simulink model "six_bots_Observer_Collision_MN_VP_NAPF"  (R2021a)
settings: Solver=ode5  StartTime=0.0  StopTime=20  FixedStep=0.005  RelTol=1e-3
(part 1 of 4)
settings Model: Creator=a1752760  LastModifiedBy=a1752760
settings SolverCC: AlgebraicLoopSolver=TrustRegion
settings DataIOCC: ReturnWorkspaceOutputs=off
settings DebuggingCC: SFMachineParentedDataDiag=warning  ArithmeticOperatorsInVariantConditions=warning
settings SFSimCC: CustomCodeUndefinedFunction=UseInterfaceOnly

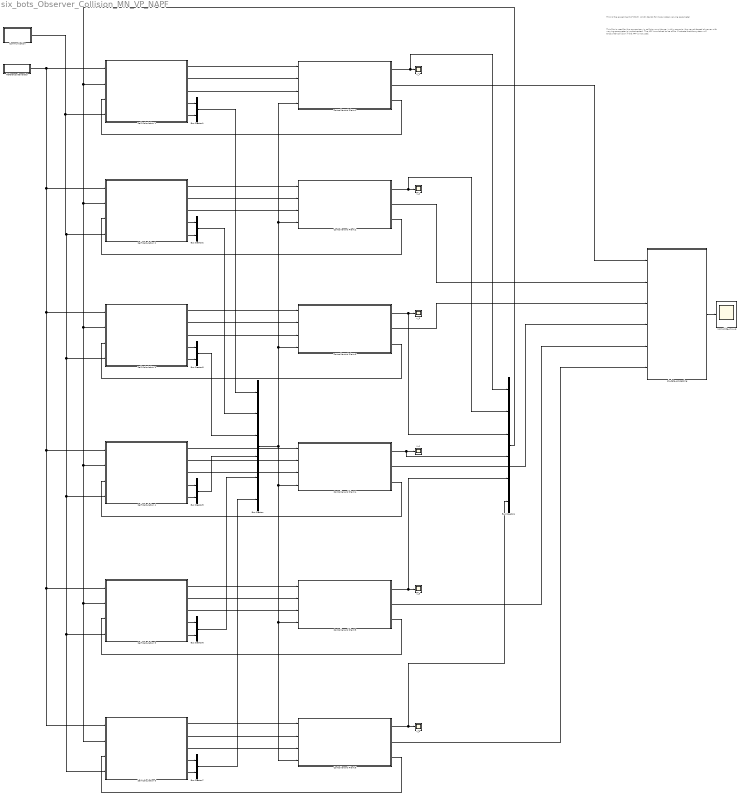
== system six_bots_Observer_Collision_MN_VP_NAPF ==
  note: This file is used for the comparison in collision avoidance. In this scenario, the neural-based
      | observer with varying-parameter is implemented. The APF is switched to be off to illustrate
      | that the system will encounter collision if the APF is not used.
  note: This is the experiment of MNVP, which stands for more nodes varying parameter
  Bus Creator : BusCreator  Inputs=6
  Bus Creator{1..3,5..7} (6 alike) : BusCreator  Inputs=2
  Bus Creator4 : BusCreator  Inputs=6
  Communication : Subsystem
  Controller and Plant 1 : Subsystem  mask{x_1=[1.8;0.1;0]}
      mask prompts: x_1 "Simulink:blkprm_prompts:IntegratorInitCond"
      mask TypeOptions x_1: x_1/InitialCondition
      mask DialogControl x_1 Prompt: Initial condition:
  Controller and Plant 2 : Subsystem  mask{x_2=[-0.9;0.6;pi/3]}
      mask prompts: x_2 "Simulink:blkprm_prompts:IntegratorInitCond"
      mask TypeOptions x_2: x_2/InitialCondition
      mask DialogControl x_2 Prompt: Initial condition:
  Controller and Plant 3 : Subsystem  mask{x_3=[-0.7;2.3;-pi/3]}
      mask prompts: x_3 "Simulink:blkprm_prompts:IntegratorInitCond"
      mask TypeOptions x_3: x_3/InitialCondition
      mask DialogControl x_3 Prompt: Initial condition:
  Controller and Plant 4 : Subsystem  mask{x_4=[0.8;-0.5;pi/2]}
      mask prompts: x_4 "Simulink:blkprm_prompts:IntegratorInitCond"
      mask TypeOptions x_4: x_4/InitialCondition
      mask DialogControl x_4 Prompt: Initial condition:
  Controller and Plant 5 : Subsystem  mask{x_5=[-0.1;-1.3;pi/4]}
      mask prompts: x_5 "Simulink:blkprm_prompts:IntegratorInitCond"
      mask TypeOptions x_5: x_5/InitialCondition
      mask DialogControl x_5 Prompt: Initial condition:
  Controller and Plant 6 : Subsystem  mask{x_6=[1.5;1.5;-pi/4]}
      mask prompts: x_6 "Simulink:blkprm_prompts:IntegratorInitCond"
      mask TypeOptions x_6: x_6/InitialCondition
      mask DialogControl x_6 Prompt: Initial condition:
  Reference Generator : Subsystem
  Self Calculation 1 : Subsystem
  Self Calculation 2 : Subsystem
  Self Calculation 3 : Subsystem
  Self Calculation 4 : Subsystem
  Self Calculation 5 : Subsystem
  Self Calculation 6 : Subsystem
  norm_tilde_mn_vp : Scope
  ob_data_processing : MATLAB Function  TreatAsAtomicUnit=on
  x_{1..6} (6 alike) : Scope
  wires:
  Controller and Plant 1/1(Position_1) -> Bus Creator4/1, x_1/1
  Controller and Plant 1/3(Control input_1) -> Self Calculation 1/3(Control Input)
  Self Calculation 1/4(delta_x) -> Bus Creator1/1
  Self Calculation 1/5(delta_v) -> Bus Creator1/2
  Self Calculation 1/1(L_i) -> Controller and Plant 1/1(L_i)
  Self Calculation 1/2(u_bar) -> Controller and Plant 1/2(u_bar)
  Self Calculation 1/3(Z_1) -> Controller and Plant 1/3(Z_1)
  Self Calculation 2/3(Z_1) -> Controller and Plant 2/3(Z_1)
  Self Calculation 2/4(delta_x) -> Bus Creator2/1
  Self Calculation 2/1(L_i) -> Controller and Plant 2/1(L_i)
  Controller and Plant 2/3(Control input_1) -> Self Calculation 2/3(Control Input)
  Self Calculation 2/2(u_bar) -> Controller and Plant 2/2(u_bar)
  Self Calculation 2/5(delta_v) -> Bus Creator2/2
  Self Calculation 3/3(Z_1) -> Controller and Plant 3/3(Z_1)
  Self Calculation 3/4(delta_x) -> Bus Creator3/1
  Self Calculation 3/1(L_i) -> Controller and Plant 3/1(L_i)
  Controller and Plant 3/3(Control input_1) -> Self Calculation 3/3(Control Input)
  Self Calculation 3/2(u_bar) -> Controller and Plant 3/2(u_bar)
  Self Calculation 3/5(delta_v) -> Bus Creator3/2
  Controller and Plant 2/1(Position_1) -> Bus Creator4/2, x_2/1
  Controller and Plant 3/1(Position_1) -> Bus Creator4/3, x_3/1
  Controller and Plant 4/3(Control input_1) -> Self Calculation 4/3(Control Input)
  Controller and Plant 4/1(Position_1) -> Bus Creator4/4, x_4/1
  Self Calculation 4/5(delta_v) -> Bus Creator5/2
  Self Calculation 4/2(u_bar) -> Controller and Plant 4/2(u_bar)
  Self Calculation 4/3(Z_1) -> Controller and Plant 4/3(Z_1)
  Self Calculation 4/4(delta_x) -> Bus Creator5/1
  Self Calculation 4/1(L_i) -> Controller and Plant 4/1(L_i)
  Controller and Plant 5/3(Control input_1) -> Self Calculation 5/3(Control Input)
  Self Calculation 5/5(delta_v) -> Bus Creator6/2
  Self Calculation 5/2(u_bar) -> Controller and Plant 5/2(u_bar)
  Self Calculation 5/3(Z_1) -> Controller and Plant 5/3(Z_1)
  Self Calculation 5/4(delta_x) -> Bus Creator6/1
  Self Calculation 5/1(L_i) -> Controller and Plant 5/1(L_i)
  Controller and Plant 6/3(Control input_1) -> Self Calculation 6/3(Control Input)
  Controller and Plant 6/1(Position_1) -> Bus Creator4/6, x_6/1
  Self Calculation 6/5(delta_v) -> Bus Creator7/2
  Self Calculation 6/2(u_bar) -> Controller and Plant 6/2(u_bar)
  Self Calculation 6/3(Z_1) -> Controller and Plant 6/3(Z_1)
  Self Calculation 6/4(delta_x) -> Bus Creator7/1
  Communication/1(Laplacian) -> Self Calculation 2/4(Laplacian), Self Calculation 6/4(Laplacian), Self Calculation 5/4(Laplacian), Self Calculation 4/4(Laplacian), Self Calculation 3/4(Laplacian), Self Calculation 1/4(Laplacian)
  Reference Generator/1(Full_reference) -> Self Calculation 2/1(Reference), Self Calculation 6/1(Reference), Self Calculation 5/1(Reference), Self Calculation 4/1(Reference), Self Calculation 3/1(Reference), Self Calculation 1/1(Reference)
  Self Calculation 6/1(L_i) -> Controller and Plant 6/1(L_i)
  Bus Creator1/1 -> Bus Creator/1
  Bus Creator2/1 -> Bus Creator/2
  Bus Creator3/1 -> Bus Creator/3
  Bus Creator5/1 -> Bus Creator/4
  Bus Creator6/1 -> Bus Creator/5
  Bus Creator7/1 -> Bus Creator/6
  Controller and Plant 5/1(Position_1) -> Bus Creator4/5, x_5/1
  Bus Creator4/1 -> Self Calculation 6/2(Position_agents), Self Calculation 5/2(Position_agents), Self Calculation 4/2(Position_agents), Self Calculation 3/2(Position_agents), Self Calculation 2/2(Position_agents), Self Calculation 1/2(Position_agents)
  Bus Creator/1 -> Controller and Plant 3/4(info_commu), Controller and Plant 2/4(info_commu), Controller and Plant 1/4(info_commu), Controller and Plant 6/4(info_commu), Controller and Plant 5/4(info_commu), Controller and Plant 4/4(info_commu)
  Controller and Plant 1/2(ob_tilde_1) -> ob_data_processing/1(ob_tilde_1)
  Controller and Plant 2/2(ob_tilde_2) -> ob_data_processing/2(ob_tilde_2)
  Controller and Plant 3/2(ob_tilde_3) -> ob_data_processing/3(ob_tilde_3)
  Controller and Plant 4/2(ob_tilde_4) -> ob_data_processing/4(ob_tilde_4)
  Controller and Plant 5/2(ob_tilde_5) -> ob_data_processing/5(ob_tilde_5)
  Controller and Plant 6/2(ob_tilde_6) -> ob_data_processing/6(ob_tilde_6)
  ob_data_processing/1(norm_tilde) -> norm_tilde_mn_vp/1

== system six_bots_Observer_Collision_MN_VP_NAPF/Communication ==
  Add : Sum
  Communication Topology : Constant  Value=[1,-1,0,0,0,0;0,1,-1,0,0,0;-1,-1,3,0,0,-1;0,0,-1,2,-1,0;0,0,0,0,1,-1;0,0,-1,-1,0,2]  VectorParams1D=off
  Constant : Constant  Value=2  VectorParams1D=off
  Product : Product
  Reference Feeding : Constant  Value=[1,0,0,0,0,0;0,1,0,0,0,0;0,0,1,0,0,0;0,0,0,1,0,0;0,0,0,0,1,0;0,0,0,0,0,1]  VectorParams1D=off
  Laplacian : Outport  VectorParamsAs1DForOutWhenUnconnected=off
  wires:
  Constant/1 -> Product/2
  Reference Feeding/1 -> Product/1
  Communication Topology/1 -> Add/1
  Product/1 -> Add/2
  Add/1 -> Laplacian/1

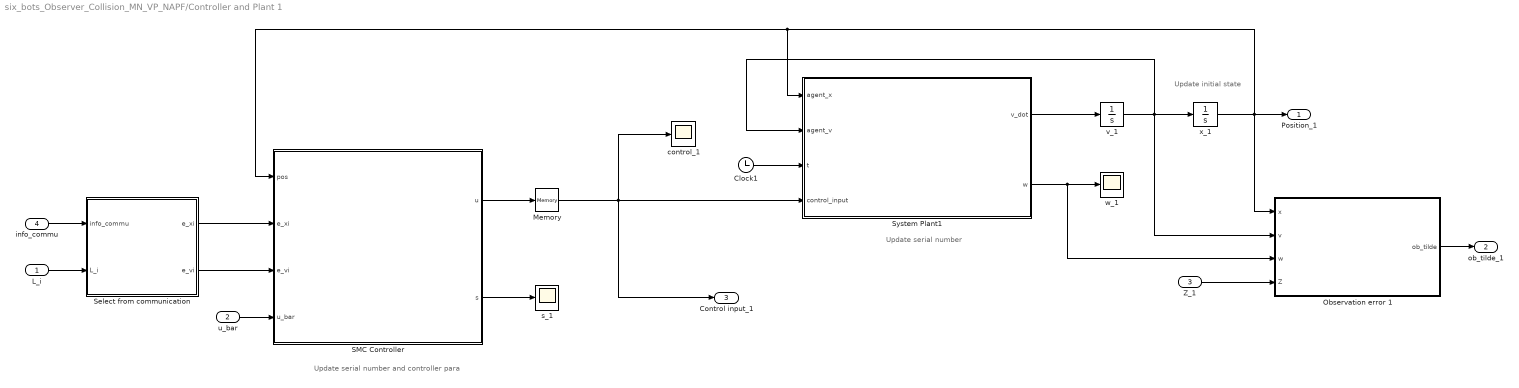
== system six_bots_Observer_Collision_MN_VP_NAPF/Controller and Plant 1 ==
  note: Update initial state
  note: Update serial number
  note: Update serial number and controller para
  L_i : Inport
  u_bar : Inport  Port=2
  Z_1 : Inport  Port=3
  info_commu : Inport  Port=4
  Clock1 : Clock
  Memory : Memory  InitialCondition=[0;0;0]
  Observation error 1 : MATLAB Function  TreatAsAtomicUnit=on
  SMC Controller : MATLAB Function  TreatAsAtomicUnit=on
  Select from communication : MATLAB Function  TreatAsAtomicUnit=on
  System Plant1 : MATLAB Function  TreatAsAtomicUnit=on
  control_1 : Scope
  s_1 : Scope
  v_1 : Integrator  InitialCondition=[0;0;0]  ContinuousStateAttributes='speed'
  w_1 : Scope
  x_1 : Integrator  Tag=Position_x1  InitialCondition=x_1  ContinuousStateAttributes='position'
  Position_1 : Outport
  ob_tilde_1 : Outport  Port=2
  Control input_1 : Outport  Port=3
  wires:
  SMC Controller/2(s) -> s_1/1
  Memory/1 -> control_1/1, System Plant1/4(control_input), Control input_1/1
  SMC Controller/1(u) -> Memory/1
  System Plant1/2(w) -> Observation error 1/3(w), w_1/1
  x_1/1 -> Observation error 1/1(x), Position_1/1, System Plant1/1(agent_x), SMC Controller/1(pos)
  v_1/1 -> Observation error 1/2(v), x_1/1, System Plant1/2(agent_v)
  System Plant1/1(v_dot) -> v_1/1
  Clock1/1 -> System Plant1/3(t)
  Select from communication/1(e_xi) -> SMC Controller/2(e_xi)
  Select from communication/2(e_vi) -> SMC Controller/3(e_vi)
  info_commu/1 -> Select from communication/1(info_commu)
  L_i/1 -> Select from communication/2(L_i)
  u_bar/1 -> SMC Controller/4(u_bar)
  Z_1/1 -> Observation error 1/4(Z)
  Observation error 1/1(ob_tilde) -> ob_tilde_1/1

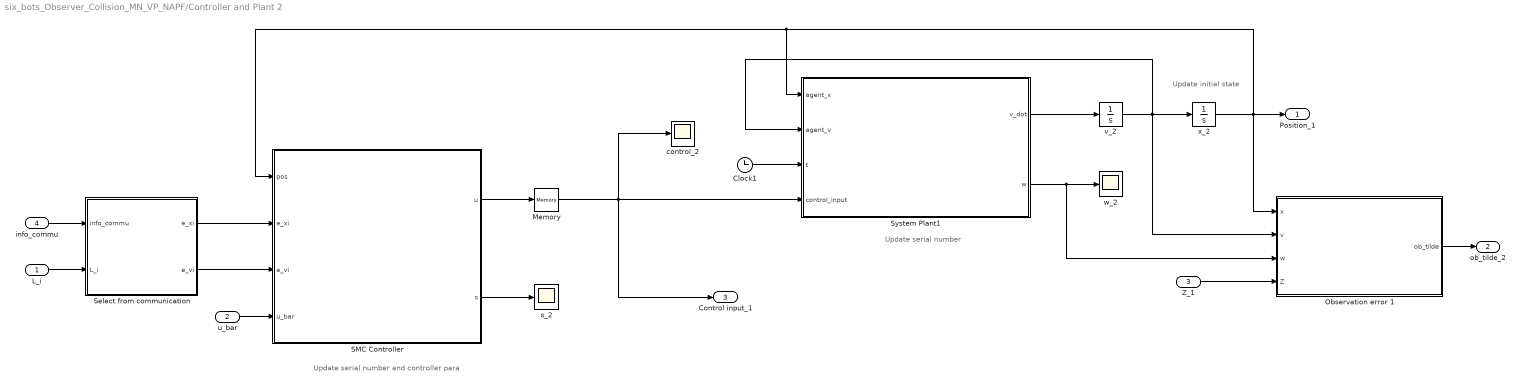
== system six_bots_Observer_Collision_MN_VP_NAPF/Controller and Plant 2 ==
  note: Update initial state
  note: Update serial number
  note: Update serial number and controller para
  L_i : Inport
  u_bar : Inport  Port=2
  Z_1 : Inport  Port=3
  info_commu : Inport  Port=4
  Clock1 : Clock
  Memory : Memory  InitialCondition=[0;0;0]
  Observation error 1 : MATLAB Function  TreatAsAtomicUnit=on
  SMC Controller : MATLAB Function  TreatAsAtomicUnit=on
  Select from communication : MATLAB Function  TreatAsAtomicUnit=on
  System Plant1 : MATLAB Function  TreatAsAtomicUnit=on
  control_2 : Scope
  s_2 : Scope
  v_2 : Integrator  InitialCondition=[0;0;0]  ContinuousStateAttributes='speed'
  w_2 : Scope
  x_2 : Integrator  Tag=Position_x1  InitialCondition=x_2  ContinuousStateAttributes='position'
  Position_1 : Outport
  ob_tilde_2 : Outport  Port=2
  Control input_1 : Outport  Port=3
  wires:
  SMC Controller/2(s) -> s_2/1
  Memory/1 -> control_2/1, System Plant1/4(control_input), Control input_1/1
  SMC Controller/1(u) -> Memory/1
  System Plant1/2(w) -> Observation error 1/3(w), w_2/1
  x_2/1 -> Observation error 1/1(x), Position_1/1, System Plant1/1(agent_x), SMC Controller/1(pos)
  v_2/1 -> Observation error 1/2(v), x_2/1, System Plant1/2(agent_v)
  System Plant1/1(v_dot) -> v_2/1
  Clock1/1 -> System Plant1/3(t)
  Select from communication/1(e_xi) -> SMC Controller/2(e_xi)
  Select from communication/2(e_vi) -> SMC Controller/3(e_vi)
  info_commu/1 -> Select from communication/1(info_commu)
  L_i/1 -> Select from communication/2(L_i)
  u_bar/1 -> SMC Controller/4(u_bar)
  Z_1/1 -> Observation error 1/4(Z)
  Observation error 1/1(ob_tilde) -> ob_tilde_2/1

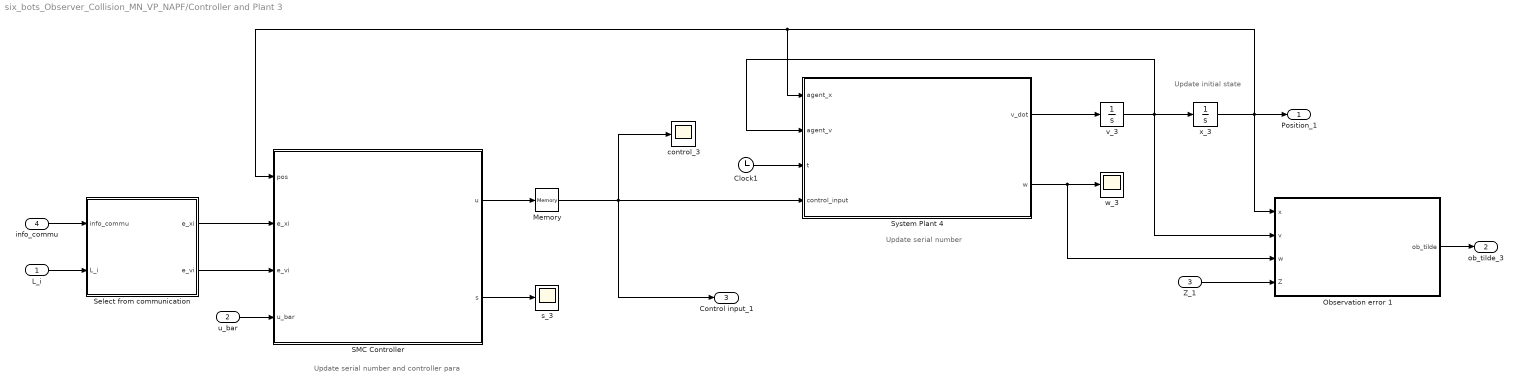
== system six_bots_Observer_Collision_MN_VP_NAPF/Controller and Plant 3 ==
  note: Update initial state
  note: Update serial number
  note: Update serial number and controller para
  L_i : Inport
  u_bar : Inport  Port=2
  Z_1 : Inport  Port=3
  info_commu : Inport  Port=4
  Clock1 : Clock
  Memory : Memory  InitialCondition=[0;0;0]
  Observation error 1 : MATLAB Function  TreatAsAtomicUnit=on
  SMC Controller : MATLAB Function  TreatAsAtomicUnit=on
  Select from communication : MATLAB Function  TreatAsAtomicUnit=on
  System Plant 4 : MATLAB Function  TreatAsAtomicUnit=on
  control_3 : Scope
  s_3 : Scope
  v_3 : Integrator  InitialCondition=[0;0;0]  ContinuousStateAttributes='speed'
  w_3 : Scope
  x_3 : Integrator  Tag=Position_x1  InitialCondition=x_3  ContinuousStateAttributes='position'
  Position_1 : Outport
  ob_tilde_3 : Outport  Port=2
  Control input_1 : Outport  Port=3
  wires:
  SMC Controller/2(s) -> s_3/1
  Memory/1 -> control_3/1, System Plant 4/4(control_input), Control input_1/1
  SMC Controller/1(u) -> Memory/1
  System Plant 4/2(w) -> Observation error 1/3(w), w_3/1
  x_3/1 -> Observation error 1/1(x), Position_1/1, System Plant 4/1(agent_x), SMC Controller/1(pos)
  v_3/1 -> Observation error 1/2(v), x_3/1, System Plant 4/2(agent_v)
  System Plant 4/1(v_dot) -> v_3/1
  Clock1/1 -> System Plant 4/3(t)
  Select from communication/1(e_xi) -> SMC Controller/2(e_xi)
  Select from communication/2(e_vi) -> SMC Controller/3(e_vi)
  info_commu/1 -> Select from communication/1(info_commu)
  L_i/1 -> Select from communication/2(L_i)
  u_bar/1 -> SMC Controller/4(u_bar)
  Z_1/1 -> Observation error 1/4(Z)
  Observation error 1/1(ob_tilde) -> ob_tilde_3/1

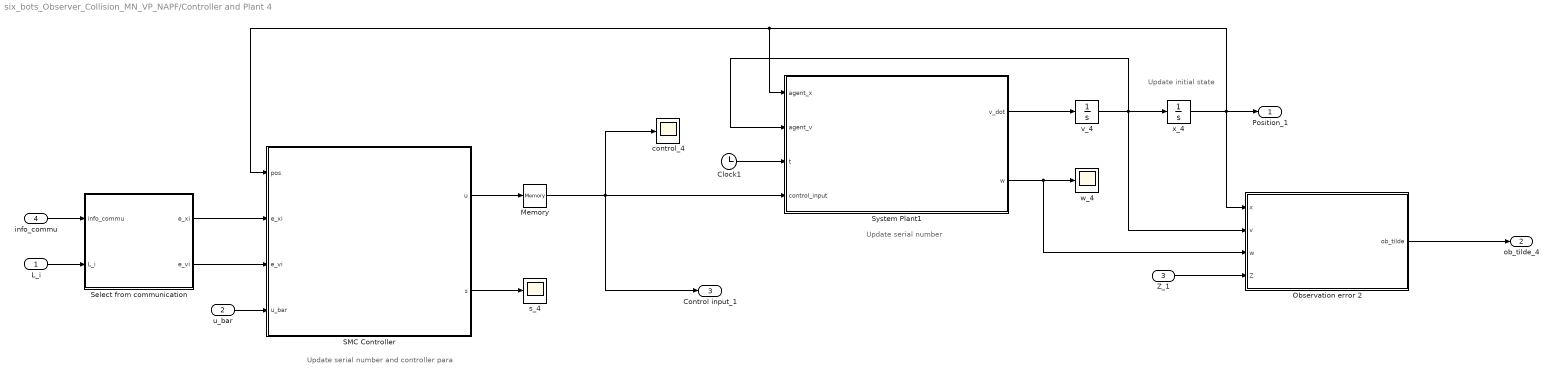
== system six_bots_Observer_Collision_MN_VP_NAPF/Controller and Plant 4 ==
  note: Update initial state
  note: Update serial number
  note: Update serial number and controller para
  L_i : Inport
  u_bar : Inport  Port=2
  Z_1 : Inport  Port=3
  info_commu : Inport  Port=4
  Clock1 : Clock
  Memory : Memory  InitialCondition=[0;0;0]
  Observation error 2 : MATLAB Function  TreatAsAtomicUnit=on
  SMC Controller : MATLAB Function  TreatAsAtomicUnit=on
  Select from communication : MATLAB Function  TreatAsAtomicUnit=on
  System Plant1 : MATLAB Function  TreatAsAtomicUnit=on
  control_4 : Scope
  s_4 : Scope
  v_4 : Integrator  InitialCondition=[0;0;0]  ContinuousStateAttributes='speed'
  w_4 : Scope
  x_4 : Integrator  Tag=Position_x1  InitialCondition=x_4  ContinuousStateAttributes='position'
  Position_1 : Outport
  ob_tilde_4 : Outport  Port=2
  Control input_1 : Outport  Port=3
  wires:
  SMC Controller/2(s) -> s_4/1
  Memory/1 -> control_4/1, System Plant1/4(control_input), Control input_1/1
  SMC Controller/1(u) -> Memory/1
  System Plant1/2(w) -> Observation error 2/3(w), w_4/1
  x_4/1 -> Observation error 2/1(x), Position_1/1, System Plant1/1(agent_x), SMC Controller/1(pos)
  v_4/1 -> Observation error 2/2(v), x_4/1, System Plant1/2(agent_v)
  System Plant1/1(v_dot) -> v_4/1
  Clock1/1 -> System Plant1/3(t)
  Select from communication/1(e_xi) -> SMC Controller/2(e_xi)
  Select from communication/2(e_vi) -> SMC Controller/3(e_vi)
  info_commu/1 -> Select from communication/1(info_commu)
  L_i/1 -> Select from communication/2(L_i)
  u_bar/1 -> SMC Controller/4(u_bar)
  Z_1/1 -> Observation error 2/4(Z)
  Observation error 2/1(ob_tilde) -> ob_tilde_4/1

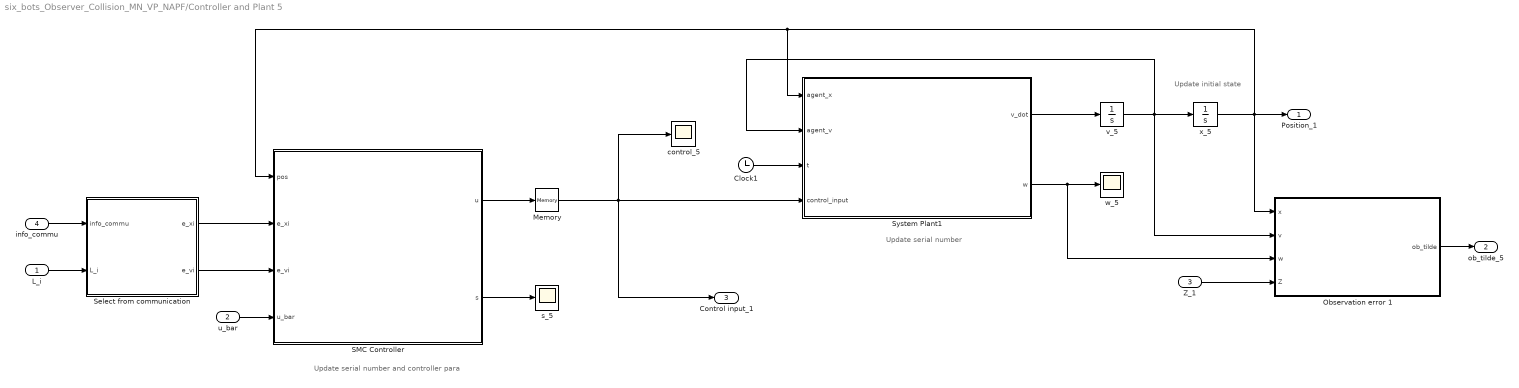
== system six_bots_Observer_Collision_MN_VP_NAPF/Controller and Plant 5 ==
  note: Update initial state
  note: Update serial number
  note: Update serial number and controller para
  L_i : Inport
  u_bar : Inport  Port=2
  Z_1 : Inport  Port=3
  info_commu : Inport  Port=4
  Clock1 : Clock
  Memory : Memory  InitialCondition=[0;0;0]
  Observation error 1 : MATLAB Function  TreatAsAtomicUnit=on
  SMC Controller : MATLAB Function  TreatAsAtomicUnit=on
  Select from communication : MATLAB Function  TreatAsAtomicUnit=on
  System Plant1 : MATLAB Function  TreatAsAtomicUnit=on
  control_5 : Scope
  s_5 : Scope
  v_5 : Integrator  InitialCondition=[0;0;0]  ContinuousStateAttributes='speed'
  w_5 : Scope
  x_5 : Integrator  Tag=Position_x1  InitialCondition=x_5  ContinuousStateAttributes='position'
  Position_1 : Outport
  ob_tilde_5 : Outport  Port=2
  Control input_1 : Outport  Port=3
  wires:
  SMC Controller/2(s) -> s_5/1
  Memory/1 -> control_5/1, System Plant1/4(control_input), Control input_1/1
  SMC Controller/1(u) -> Memory/1
  System Plant1/2(w) -> Observation error 1/3(w), w_5/1
  x_5/1 -> Observation error 1/1(x), Position_1/1, System Plant1/1(agent_x), SMC Controller/1(pos)
  v_5/1 -> Observation error 1/2(v), x_5/1, System Plant1/2(agent_v)
  System Plant1/1(v_dot) -> v_5/1
  Clock1/1 -> System Plant1/3(t)
  Select from communication/1(e_xi) -> SMC Controller/2(e_xi)
  Select from communication/2(e_vi) -> SMC Controller/3(e_vi)
  info_commu/1 -> Select from communication/1(info_commu)
  L_i/1 -> Select from communication/2(L_i)
  u_bar/1 -> SMC Controller/4(u_bar)
  Z_1/1 -> Observation error 1/4(Z)
  Observation error 1/1(ob_tilde) -> ob_tilde_5/1

== system six_bots_Observer_Collision_MN_VP_NAPF/Controller and Plant 6 ==
  note: Update initial state
  note: Update serial number
  note: Update serial number and controller para
  L_i : Inport
  u_bar : Inport  Port=2
  Z_1 : Inport  Port=3
  info_commu : Inport  Port=4
  Clock1 : Clock
  Memory : Memory  InitialCondition=[0;0;0]
  Observation error 1 : MATLAB Function  TreatAsAtomicUnit=on
  SMC Controller : MATLAB Function  TreatAsAtomicUnit=on
  Select from communication : MATLAB Function  TreatAsAtomicUnit=on
  System Plant1 : MATLAB Function  TreatAsAtomicUnit=on
  control_6 : Scope
  s_6 : Scope
  v_6 : Integrator  InitialCondition=[0;0;0]  ContinuousStateAttributes='speed'
  w_6 : Scope
  x_6 : Integrator  Tag=Position_x1  InitialCondition=x_6  ContinuousStateAttributes='position'
  Position_1 : Outport
  ob_tilde_6 : Outport  Port=2
  Control input_1 : Outport  Port=3
  wires:
  SMC Controller/2(s) -> s_6/1
  Memory/1 -> control_6/1, System Plant1/4(control_input), Control input_1/1
  SMC Controller/1(u) -> Memory/1
  System Plant1/2(w) -> Observation error 1/3(w), w_6/1
  x_6/1 -> Observation error 1/1(x), Position_1/1, System Plant1/1(agent_x), SMC Controller/1(pos)
  v_6/1 -> Observation error 1/2(v), x_6/1, System Plant1/2(agent_v)
  System Plant1/1(v_dot) -> v_6/1
  Clock1/1 -> System Plant1/3(t)
  Select from communication/1(e_xi) -> SMC Controller/2(e_xi)
  Select from communication/2(e_vi) -> SMC Controller/3(e_vi)
  info_commu/1 -> Select from communication/1(info_commu)
  L_i/1 -> Select from communication/2(L_i)
  u_bar/1 -> SMC Controller/4(u_bar)
  Z_1/1 -> Observation error 1/4(Z)
  Observation error 1/1(ob_tilde) -> ob_tilde_6/1

== system six_bots_Observer_Collision_MN_VP_NAPF/Reference Generator ==
  Clock : Clock
  Position Reference : MATLAB Function  TreatAsAtomicUnit=on
  Position_ref : Scope
  Full_reference : Outport  VectorParamsAs1DForOutWhenUnconnected=off
  wires:
  Clock/1 -> Position Reference/1(t)
  Position Reference/1(x1d) -> Full_reference/1, Position_ref/1

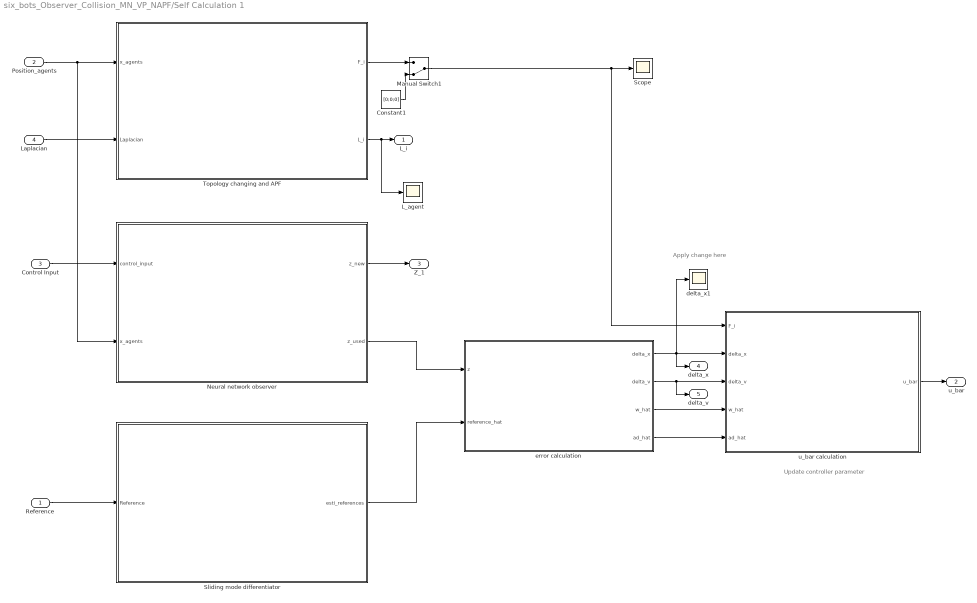
== system six_bots_Observer_Collision_MN_VP_NAPF/Self Calculation 1 ==
  note: Update controller parameter
  note: Apply change here
  Reference : Inport
  Position_agents : Inport  Port=2
  Control Input : Inport  Port=3
  Laplacian : Inport  Port=4
  Constant1 : Constant  Value=[0;0;0]  VectorParams1D=off
  L_agent : Scope
  Manual Switch1 : ManualSwitch  CurrentSetting=0
  Neural network observer : Subsystem
  Scope : Scope
  Sliding mode differentiator : Subsystem
  Topology changing and APF : Subsystem
  delta_x1 : Scope
  error calculation : MATLAB Function  TreatAsAtomicUnit=on
  u_bar calculation : MATLAB Function  TreatAsAtomicUnit=on
  L_i : Outport
  u_bar : Outport  Port=2
  Z_1 : Outport  Port=3
  delta_x : Outport  Port=4
  delta_v : Outport  Port=5
  wires:
  Manual Switch1/1 -> u_bar calculation/1(F_i), Scope/1
  Topology changing and APF/1(F_i) -> Manual Switch1/1
  Constant1/1 -> Manual Switch1/2
  Position_agents/1 -> Neural network observer/2(x_agents), Topology changing and APF/1(x_agents)
  Laplacian/1 -> Topology changing and APF/2("Laplacian ")
  Control Input/1 -> Neural network observer/1(control_input)
  Reference/1 -> Sliding mode differentiator/1(Reference)
  Sliding mode differentiator/1(esti_references) -> error calculation/2(reference_hat)
  error calculation/1(delta_x) -> delta_x1/1, delta_x/1, u_bar calculation/2(delta_x)
  error calculation/2(delta_v) -> delta_v/1, u_bar calculation/3(delta_v)
  error calculation/3(w_hat) -> u_bar calculation/4(w_hat)
  error calculation/4(ad_hat) -> u_bar calculation/5(ad_hat)
  u_bar calculation/1(u_bar) -> u_bar/1
  Neural network observer/2(z_used) -> error calculation/1(z)
  Neural network observer/1(z_new) -> Z_1/1
  Topology changing and APF/2(L_i) -> L_agent/1, L_i/1

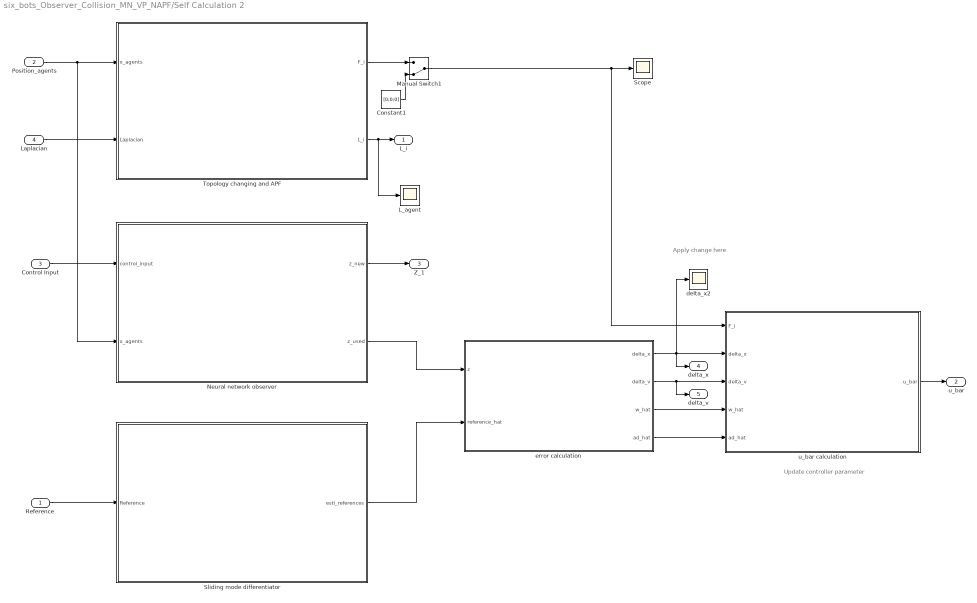
== system six_bots_Observer_Collision_MN_VP_NAPF/Self Calculation 2 ==
  note: Update controller parameter
  note: Apply change here
  Reference : Inport
  Position_agents : Inport  Port=2
  Control Input : Inport  Port=3
  Laplacian : Inport  Port=4
  Constant1 : Constant  Value=[0;0;0]  VectorParams1D=off
  L_agent : Scope
  Manual Switch1 : ManualSwitch  CurrentSetting=0
  Neural network observer : Subsystem
  Scope : Scope
  Sliding mode differentiator : Subsystem
  Topology changing and APF : Subsystem
  delta_x2 : Scope
  error calculation : MATLAB Function  TreatAsAtomicUnit=on
  u_bar calculation : MATLAB Function  TreatAsAtomicUnit=on
  L_i : Outport
  u_bar : Outport  Port=2
  Z_1 : Outport  Port=3
  delta_x : Outport  Port=4
  delta_v : Outport  Port=5
  wires:
  Manual Switch1/1 -> u_bar calculation/1(F_i), Scope/1
  Topology changing and APF/1(F_i) -> Manual Switch1/1
  Constant1/1 -> Manual Switch1/2
  Position_agents/1 -> Neural network observer/2(x_agents), Topology changing and APF/1(x_agents)
  Laplacian/1 -> Topology changing and APF/2("Laplacian ")
  Control Input/1 -> Neural network observer/1(control_input)
  Reference/1 -> Sliding mode differentiator/1(Reference)
  Sliding mode differentiator/1(esti_references) -> error calculation/2(reference_hat)
  error calculation/1(delta_x) -> delta_x2/1, delta_x/1, u_bar calculation/2(delta_x)
  error calculation/2(delta_v) -> delta_v/1, u_bar calculation/3(delta_v)
  error calculation/3(w_hat) -> u_bar calculation/4(w_hat)
  error calculation/4(ad_hat) -> u_bar calculation/5(ad_hat)
  u_bar calculation/1(u_bar) -> u_bar/1
  Neural network observer/2(z_used) -> error calculation/1(z)
  Neural network observer/1(z_new) -> Z_1/1
  Topology changing and APF/2(L_i) -> L_agent/1, L_i/1

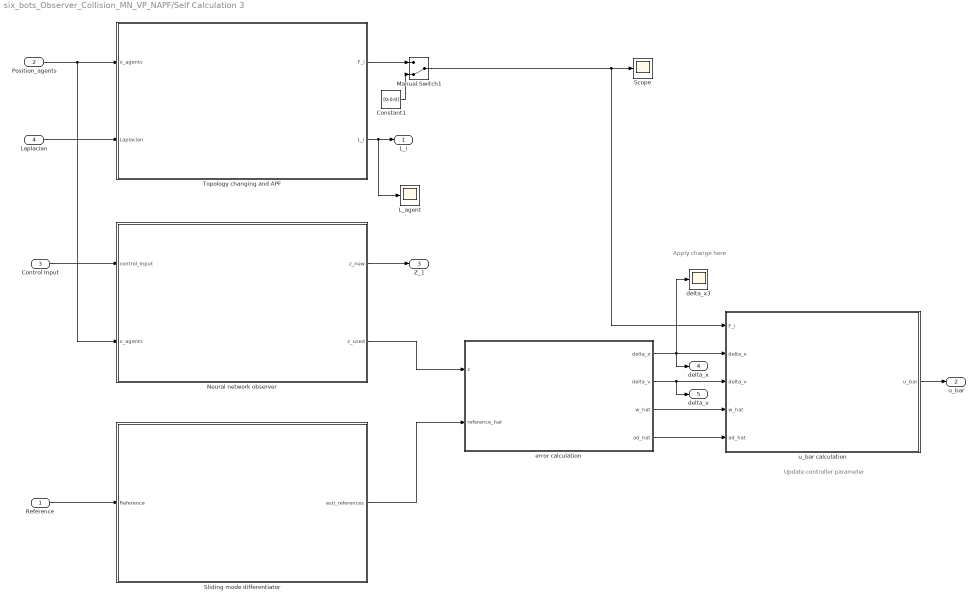
== system six_bots_Observer_Collision_MN_VP_NAPF/Self Calculation 3 ==
  note: Update controller parameter
  note: Apply change here
  Reference : Inport
  Position_agents : Inport  Port=2
  Control Input : Inport  Port=3
  Laplacian : Inport  Port=4
  Constant1 : Constant  Value=[0;0;0]  VectorParams1D=off
  L_agent : Scope
  Manual Switch1 : ManualSwitch  CurrentSetting=0
  Neural network observer : Subsystem
  Scope : Scope
  Sliding mode differentiator : Subsystem
  Topology changing and APF : Subsystem
  delta_x3 : Scope
  error calculation : MATLAB Function  TreatAsAtomicUnit=on
  u_bar calculation : MATLAB Function  TreatAsAtomicUnit=on
  L_i : Outport
  u_bar : Outport  Port=2
  Z_1 : Outport  Port=3
  delta_x : Outport  Port=4
  delta_v : Outport  Port=5
  wires:
  Manual Switch1/1 -> u_bar calculation/1(F_i), Scope/1
  Topology changing and APF/1(F_i) -> Manual Switch1/1
  Constant1/1 -> Manual Switch1/2
  Position_agents/1 -> Neural network observer/2(x_agents), Topology changing and APF/1(x_agents)
  Laplacian/1 -> Topology changing and APF/2("Laplacian ")
  Control Input/1 -> Neural network observer/1(control_input)
  Reference/1 -> Sliding mode differentiator/1(Reference)
  Sliding mode differentiator/1(esti_references) -> error calculation/2(reference_hat)
  error calculation/1(delta_x) -> delta_x3/1, delta_x/1, u_bar calculation/2(delta_x)
  error calculation/2(delta_v) -> delta_v/1, u_bar calculation/3(delta_v)
  error calculation/3(w_hat) -> u_bar calculation/4(w_hat)
  error calculation/4(ad_hat) -> u_bar calculation/5(ad_hat)
  u_bar calculation/1(u_bar) -> u_bar/1
  Neural network observer/2(z_used) -> error calculation/1(z)
  Neural network observer/1(z_new) -> Z_1/1
  Topology changing and APF/2(L_i) -> L_agent/1, L_i/1

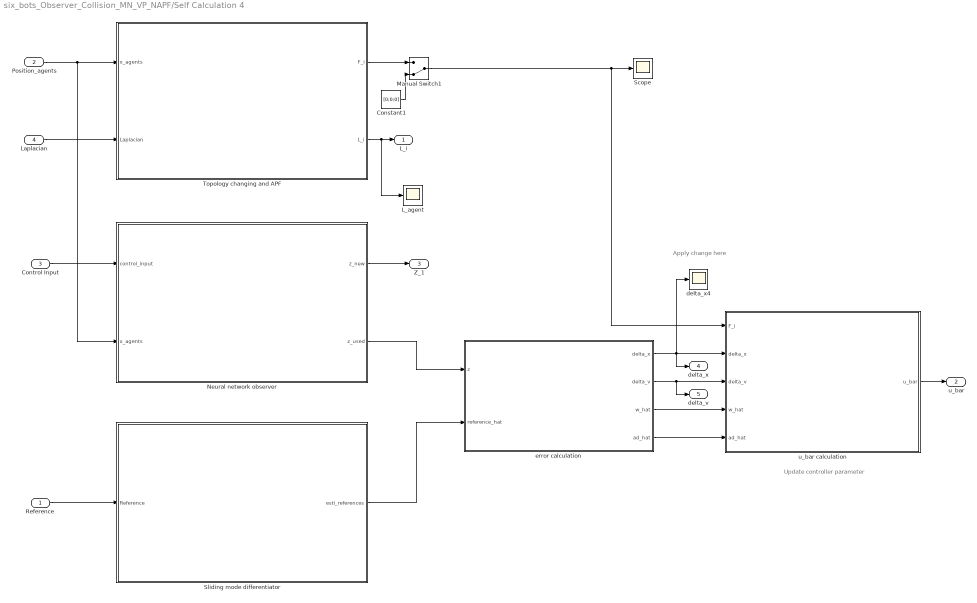
== system six_bots_Observer_Collision_MN_VP_NAPF/Self Calculation 4 ==
  note: Update controller parameter
  note: Apply change here
  Reference : Inport
  Position_agents : Inport  Port=2
  Control Input : Inport  Port=3
  Laplacian : Inport  Port=4
  Constant1 : Constant  Value=[0;0;0]  VectorParams1D=off
  L_agent : Scope
  Manual Switch1 : ManualSwitch  CurrentSetting=0
  Neural network observer : Subsystem
  Scope : Scope
  Sliding mode differentiator : Subsystem
  Topology changing and APF : Subsystem
  delta_x4 : Scope
  error calculation : MATLAB Function  TreatAsAtomicUnit=on
  u_bar calculation : MATLAB Function  TreatAsAtomicUnit=on
  L_i : Outport
  u_bar : Outport  Port=2
  Z_1 : Outport  Port=3
  delta_x : Outport  Port=4
  delta_v : Outport  Port=5
  wires:
  Manual Switch1/1 -> u_bar calculation/1(F_i), Scope/1
  Topology changing and APF/1(F_i) -> Manual Switch1/1
  Constant1/1 -> Manual Switch1/2
  Position_agents/1 -> Neural network observer/2(x_agents), Topology changing and APF/1(x_agents)
  Laplacian/1 -> Topology changing and APF/2("Laplacian ")
  Control Input/1 -> Neural network observer/1(control_input)
  Reference/1 -> Sliding mode differentiator/1(Reference)
  Sliding mode differentiator/1(esti_references) -> error calculation/2(reference_hat)
  error calculation/1(delta_x) -> delta_x4/1, delta_x/1, u_bar calculation/2(delta_x)
  error calculation/2(delta_v) -> delta_v/1, u_bar calculation/3(delta_v)
  error calculation/3(w_hat) -> u_bar calculation/4(w_hat)
  error calculation/4(ad_hat) -> u_bar calculation/5(ad_hat)
  u_bar calculation/1(u_bar) -> u_bar/1
  Neural network observer/2(z_used) -> error calculation/1(z)
  Neural network observer/1(z_new) -> Z_1/1
  Topology changing and APF/2(L_i) -> L_agent/1, L_i/1

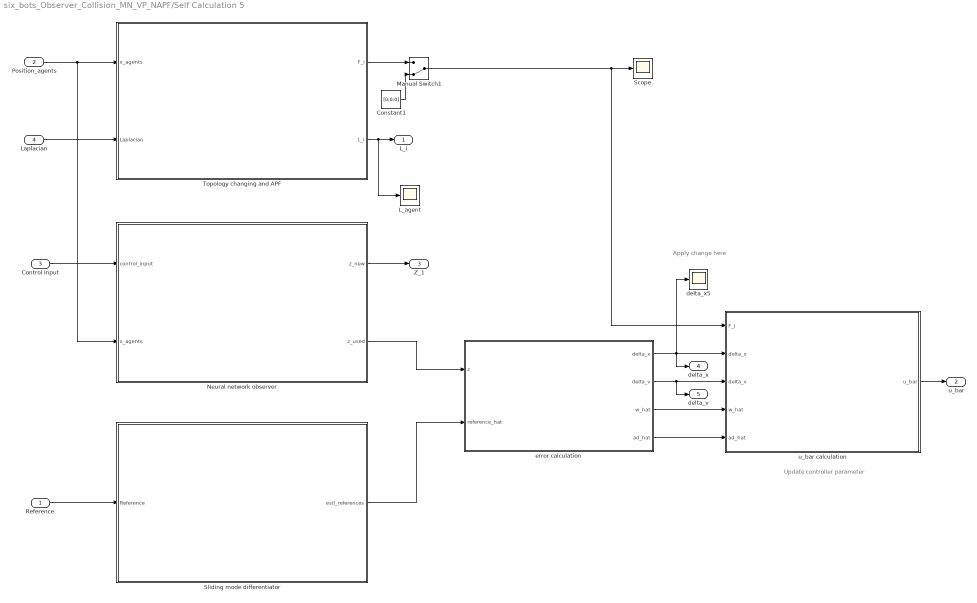
== system six_bots_Observer_Collision_MN_VP_NAPF/Self Calculation 5 ==
  note: Update controller parameter
  note: Apply change here
  Reference : Inport
  Position_agents : Inport  Port=2
  Control Input : Inport  Port=3
  Laplacian : Inport  Port=4
  Constant1 : Constant  Value=[0;0;0]  VectorParams1D=off
  L_agent : Scope
  Manual Switch1 : ManualSwitch  CurrentSetting=0
  Neural network observer : Subsystem
  Scope : Scope
  Sliding mode differentiator : Subsystem
  Topology changing and APF : Subsystem
  delta_x5 : Scope
  error calculation : MATLAB Function  TreatAsAtomicUnit=on
  u_bar calculation : MATLAB Function  TreatAsAtomicUnit=on
  L_i : Outport
  u_bar : Outport  Port=2
  Z_1 : Outport  Port=3
  delta_x : Outport  Port=4
  delta_v : Outport  Port=5
  wires:
  Manual Switch1/1 -> u_bar calculation/1(F_i), Scope/1
  Topology changing and APF/1(F_i) -> Manual Switch1/1
  Constant1/1 -> Manual Switch1/2
  Position_agents/1 -> Neural network observer/2(x_agents), Topology changing and APF/1(x_agents)
  Laplacian/1 -> Topology changing and APF/2("Laplacian ")
  Control Input/1 -> Neural network observer/1(control_input)
  Reference/1 -> Sliding mode differentiator/1(Reference)
  Sliding mode differentiator/1(esti_references) -> error calculation/2(reference_hat)
  error calculation/1(delta_x) -> delta_x5/1, delta_x/1, u_bar calculation/2(delta_x)
  error calculation/2(delta_v) -> delta_v/1, u_bar calculation/3(delta_v)
  error calculation/3(w_hat) -> u_bar calculation/4(w_hat)
  error calculation/4(ad_hat) -> u_bar calculation/5(ad_hat)
  u_bar calculation/1(u_bar) -> u_bar/1
  Neural network observer/2(z_used) -> error calculation/1(z)
  Neural network observer/1(z_new) -> Z_1/1
  Topology changing and APF/2(L_i) -> L_agent/1, L_i/1

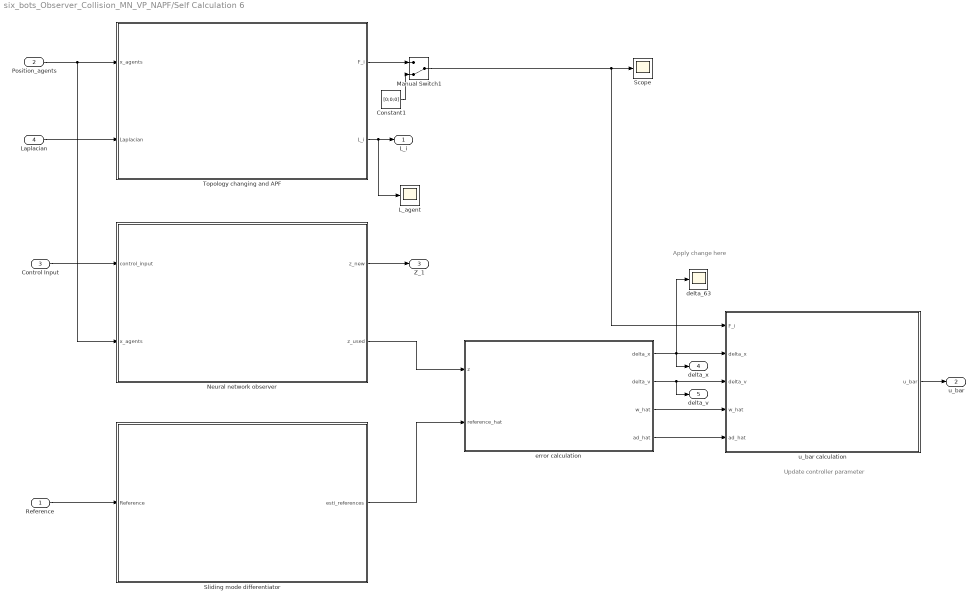
== system six_bots_Observer_Collision_MN_VP_NAPF/Self Calculation 6 ==
  note: Update controller parameter
  note: Apply change here
  Reference : Inport
  Position_agents : Inport  Port=2
  Control Input : Inport  Port=3
  Laplacian : Inport  Port=4
  Constant1 : Constant  Value=[0;0;0]  VectorParams1D=off
  L_agent : Scope
  Manual Switch1 : ManualSwitch  CurrentSetting=0
  Neural network observer : Subsystem
  Scope : Scope
  Sliding mode differentiator : Subsystem
  Topology changing and APF : Subsystem
  delta_63 : Scope
  error calculation : MATLAB Function  TreatAsAtomicUnit=on
  u_bar calculation : MATLAB Function  TreatAsAtomicUnit=on
  L_i : Outport
  u_bar : Outport  Port=2
  Z_1 : Outport  Port=3
  delta_x : Outport  Port=4
  delta_v : Outport  Port=5
  wires:
  Manual Switch1/1 -> u_bar calculation/1(F_i), Scope/1
  Topology changing and APF/1(F_i) -> Manual Switch1/1
  Constant1/1 -> Manual Switch1/2
  Position_agents/1 -> Neural network observer/2(x_agents), Topology changing and APF/1(x_agents)
  Laplacian/1 -> Topology changing and APF/2("Laplacian ")
  Control Input/1 -> Neural network observer/1(control_input)
  Reference/1 -> Sliding mode differentiator/1(Reference)
  Sliding mode differentiator/1(esti_references) -> error calculation/2(reference_hat)
  error calculation/1(delta_x) -> delta_63/1, delta_x/1, u_bar calculation/2(delta_x)
  error calculation/2(delta_v) -> delta_v/1, u_bar calculation/3(delta_v)
  error calculation/3(w_hat) -> u_bar calculation/4(w_hat)
  error calculation/4(ad_hat) -> u_bar calculation/5(ad_hat)
  u_bar calculation/1(u_bar) -> u_bar/1
  Neural network observer/2(z_used) -> error calculation/1(z)
  Neural network observer/1(z_new) -> Z_1/1
  Topology changing and APF/2(L_i) -> L_agent/1, L_i/1

== system six_bots_Observer_Collision_MN_VP_NAPF/Self Calculation 1/Neural network observer ==
  note: Update serial number
  note: Update serial number
  control_input : Inport
  x_agents : Inport  Port=2
  Finite observer : Subsystem
  Position selection : MATLAB Function  TreatAsAtomicUnit=on
  z_new : Outport
  z_used : Outport  Port=2
  wires:
  control_input/1 -> Finite observer/1(u)
  Position selection/1(x_agent) -> Finite observer/2(x)
  x_agents/1 -> Position selection/1(x_agents)
  Finite observer/1(z_new) -> z_new/1
  Finite observer/2(z_used) -> z_used/1

== system six_bots_Observer_Collision_MN_VP_NAPF/Self Calculation 1/Sliding mode differentiator ==
  note: Update serial number
  note: Update initial state
  Reference : Inport
  Integrator : Integrator  InitialCondition=[0.7;1.7;0;0;0;0;0;0;0;0;0;0]  ContinuousStateAttributes='speed'
  MATLAB Function : MATLAB Function  TreatAsAtomicUnit=on
  Reference selection : MATLAB Function  TreatAsAtomicUnit=on
  sliding mode differentiator : MATLAB Function  TreatAsAtomicUnit=on
  esti_references : Outport
  wires:
  Reference/1 -> Reference selection/1(reference)
  sliding mode differentiator/1(z_dot) -> Integrator/1
  MATLAB Function/1(esti_references) -> esti_references/1
  Reference selection/1(agent_reference) -> MATLAB Function/2(x_d), sliding mode differentiator/2(x_d)
  Integrator/1 -> MATLAB Function/1(z), sliding mode differentiator/1(z)

== system six_bots_Observer_Collision_MN_VP_NAPF/Self Calculation 1/Topology changing and APF ==
  note: Update topology parameters
  note: Update APF parameter
  note: Apply change here
  x_agents : Inport
  "Laplacian " : Inport  Port=2
  Changing topology : MATLAB Function  TreatAsAtomicUnit=on
  Communication based APF : MATLAB Function  TreatAsAtomicUnit=on
  rel_distance_1 : Scope
  F_i : Outport
  L_i : Outport  Port=2
  wires:
  x_agents/1 -> Communication based APF/1(x_agents), Changing topology/1(x_agents)
  "Laplacian "/1 -> Changing topology/2(L)
  Changing topology/1(rel_distance) -> rel_distance_1/1
  Changing topology/2(L_i) -> L_i/1, Communication based APF/2(L_i)
  Communication based APF/1(F_i) -> F_i/1

== system six_bots_Observer_Collision_MN_VP_NAPF/Self Calculation 2/Neural network observer ==
  note: Update serial number
  note: Update serial number
  control_input : Inport
  x_agents : Inport  Port=2
  Finite observer : Subsystem
  Position selection : MATLAB Function  TreatAsAtomicUnit=on
  z_new : Outport
  z_used : Outport  Port=2
  wires:
  control_input/1 -> Finite observer/1(u)
  Position selection/1(x_agent) -> Finite observer/2(x)
  x_agents/1 -> Position selection/1(x_agents)
  Finite observer/1(z_new) -> z_new/1
  Finite observer/2(z_used) -> z_used/1

== system six_bots_Observer_Collision_MN_VP_NAPF/Self Calculation 2/Sliding mode differentiator ==
  note: Update serial number
  note: Update initial state
  Reference : Inport
  Integrator : Integrator  InitialCondition=[-1;1.4;0;0;0;0;0;0;0;0;0;0]  ContinuousStateAttributes='speed'
  MATLAB Function : MATLAB Function  TreatAsAtomicUnit=on
  Reference selection : MATLAB Function  TreatAsAtomicUnit=on
  sliding mode differentiator : MATLAB Function  TreatAsAtomicUnit=on
  esti_references : Outport
  wires:
  Reference/1 -> Reference selection/1(reference)
  sliding mode differentiator/1(z_dot) -> Integrator/1
  MATLAB Function/1(esti_references) -> esti_references/1
  Reference selection/1(agent_reference) -> MATLAB Function/2(x_d), sliding mode differentiator/2(x_d)
  Integrator/1 -> MATLAB Function/1(z), sliding mode differentiator/1(z)

== system six_bots_Observer_Collision_MN_VP_NAPF/Self Calculation 2/Topology changing and APF ==
  note: Apply change here
  note: Update topology parameters
  note: Update APF parameter
  x_agents : Inport
  "Laplacian " : Inport  Port=2
  Changing topology : MATLAB Function  TreatAsAtomicUnit=on
  Communication based APF : MATLAB Function  TreatAsAtomicUnit=on
  rel_distance_2 : Scope
  F_i : Outport
  L_i : Outport  Port=2
  wires:
  x_agents/1 -> Communication based APF/1(x_agents), Changing topology/1(x_agents)
  "Laplacian "/1 -> Changing topology/2(L)
  Changing topology/1(rel_distance) -> rel_distance_2/1
  Changing topology/2(L_i) -> L_i/1, Communication based APF/2(L_i)
  Communication based APF/1(F_i) -> F_i/1

== system six_bots_Observer_Collision_MN_VP_NAPF/Self Calculation 3/Neural network observer ==
  note: Update serial number
  note: Update serial number
  control_input : Inport
  x_agents : Inport  Port=2
  Finite observer : Subsystem
  Position selection : MATLAB Function  TreatAsAtomicUnit=on
  z_new : Outport
  z_used : Outport  Port=2
  wires:
  control_input/1 -> Finite observer/1(u)
  Position selection/1(x_agent) -> Finite observer/2(x)
  x_agents/1 -> Position selection/1(x_agents)
  Finite observer/1(z_new) -> z_new/1
  Finite observer/2(z_used) -> z_used/1

== system six_bots_Observer_Collision_MN_VP_NAPF/Self Calculation 3/Sliding mode differentiator ==
  note: Update serial number
  note: Update initial state
  Reference : Inport
  Integrator : Integrator  InitialCondition=[-1.6;0.2;0;0;0;0;0;0;0;0;0;0]  ContinuousStateAttributes='speed'
  MATLAB Function : MATLAB Function  TreatAsAtomicUnit=on
  Reference selection : MATLAB Function  TreatAsAtomicUnit=on
  sliding mode differentiator : MATLAB Function  TreatAsAtomicUnit=on
  esti_references : Outport
  wires:
  Reference/1 -> Reference selection/1(reference)
  sliding mode differentiator/1(z_dot) -> Integrator/1
  MATLAB Function/1(esti_references) -> esti_references/1
  Reference selection/1(agent_reference) -> MATLAB Function/2(x_d), sliding mode differentiator/2(x_d)
  Integrator/1 -> MATLAB Function/1(z), sliding mode differentiator/1(z)

== system six_bots_Observer_Collision_MN_VP_NAPF/Self Calculation 3/Topology changing and APF ==
  note: Apply change here
  note: Update topology parameters
  note: Update APF parameter
  x_agents : Inport
  "Laplacian " : Inport  Port=2
  Changing topology : MATLAB Function  TreatAsAtomicUnit=on
  Communication based APF : MATLAB Function  TreatAsAtomicUnit=on
  rel_distance_3 : Scope
  F_i : Outport
  L_i : Outport  Port=2
  wires:
  x_agents/1 -> Communication based APF/1(x_agents), Changing topology/1(x_agents)
  "Laplacian "/1 -> Changing topology/2(L)
  Changing topology/1(rel_distance) -> rel_distance_3/1
  Changing topology/2(L_i) -> L_i/1, Communication based APF/2(L_i)
  Communication based APF/1(F_i) -> F_i/1

== system six_bots_Observer_Collision_MN_VP_NAPF/Self Calculation 4/Neural network observer ==
  note: Update serial number
  note: Update serial number
  control_input : Inport
  x_agents : Inport  Port=2
  Finite observer : Subsystem
  Position selection : MATLAB Function  TreatAsAtomicUnit=on
  z_new : Outport
  z_used : Outport  Port=2
  wires:
  control_input/1 -> Finite observer/1(u)
  Position selection/1(x_agent) -> Finite observer/2(x)
  x_agents/1 -> Position selection/1(x_agents)
  Finite observer/1(z_new) -> z_new/1
  Finite observer/2(z_used) -> z_used/1

== system six_bots_Observer_Collision_MN_VP_NAPF/Self Calculation 4/Sliding mode differentiator ==
  note: Update serial number
  note: Update initial state
  Reference : Inport
  Integrator : Integrator  InitialCondition=[-1.1;-1.3;0;0;0;0;0;0;0;0;0;0]  ContinuousStateAttributes='speed'
  MATLAB Function : MATLAB Function  TreatAsAtomicUnit=on
  Reference selection : MATLAB Function  TreatAsAtomicUnit=on
  sliding mode differentiator : MATLAB Function  TreatAsAtomicUnit=on
  esti_references : Outport
  wires:
  Reference/1 -> Reference selection/1(reference)
  sliding mode differentiator/1(z_dot) -> Integrator/1
  MATLAB Function/1(esti_references) -> esti_references/1
  Reference selection/1(agent_reference) -> MATLAB Function/2(x_d), sliding mode differentiator/2(x_d)
  Integrator/1 -> MATLAB Function/1(z), sliding mode differentiator/1(z)

== system six_bots_Observer_Collision_MN_VP_NAPF/Self Calculation 4/Topology changing and APF ==
  note: Apply change here
  note: Update topology parameters
  note: Update APF parameter
  x_agents : Inport
  "Laplacian " : Inport  Port=2
  Changing topology : MATLAB Function  TreatAsAtomicUnit=on
  Communication based APF : MATLAB Function  TreatAsAtomicUnit=on
  rel_distance_4 : Scope
  F_i : Outport
  L_i : Outport  Port=2
  wires:
  x_agents/1 -> Communication based APF/1(x_agents), Changing topology/1(x_agents)
  "Laplacian "/1 -> Changing topology/2(L)
  Changing topology/1(rel_distance) -> rel_distance_4/1
  Changing topology/2(L_i) -> L_i/1, Communication based APF/2(L_i)
  Communication based APF/1(F_i) -> F_i/1

== system six_bots_Observer_Collision_MN_VP_NAPF/Self Calculation 5/Neural network observer ==
  note: Update serial number
  note: Update serial number
  control_input : Inport
  x_agents : Inport  Port=2
  Finite observer : Subsystem
  Position selection : MATLAB Function  TreatAsAtomicUnit=on
  z_new : Outport
  z_used : Outport  Port=2
  wires:
  control_input/1 -> Finite observer/1(u)
  Position selection/1(x_agent) -> Finite observer/2(x)
  x_agents/1 -> Position selection/1(x_agents)
  Finite observer/1(z_new) -> z_new/1
  Finite observer/2(z_used) -> z_used/1

== system six_bots_Observer_Collision_MN_VP_NAPF/Self Calculation 5/Sliding mode differentiator ==
  note: Update serial number
  note: Update initial state
  Reference : Inport
  Integrator : Integrator  InitialCondition=[0.7;-1.7;0;0;0;0;0;0;0;0;0;0]  ContinuousStateAttributes='speed'
  MATLAB Function : MATLAB Function  TreatAsAtomicUnit=on
  Reference selection : MATLAB Function  TreatAsAtomicUnit=on
  sliding mode differentiator : MATLAB Function  TreatAsAtomicUnit=on
  esti_references : Outport
  wires:
  Reference/1 -> Reference selection/1(reference)
  sliding mode differentiator/1(z_dot) -> Integrator/1
  MATLAB Function/1(esti_references) -> esti_references/1
  Reference selection/1(agent_reference) -> MATLAB Function/2(x_d), sliding mode differentiator/2(x_d)
  Integrator/1 -> MATLAB Function/1(z), sliding mode differentiator/1(z)

== system six_bots_Observer_Collision_MN_VP_NAPF/Self Calculation 5/Topology changing and APF ==
  note: Apply change here
  note: Update topology parameters
  note: Update APF parameter
  x_agents : Inport
  "Laplacian " : Inport  Port=2
  Changing topology : MATLAB Function  TreatAsAtomicUnit=on
  Communication based APF : MATLAB Function  TreatAsAtomicUnit=on
  rel_distance_5 : Scope
  F_i : Outport
  L_i : Outport  Port=2
  wires:
  x_agents/1 -> Communication based APF/1(x_agents), Changing topology/1(x_agents)
  "Laplacian "/1 -> Changing topology/2(L)
  Changing topology/1(rel_distance) -> rel_distance_5/1
  Changing topology/2(L_i) -> L_i/1, Communication based APF/2(L_i)
  Communication based APF/1(F_i) -> F_i/1

== system six_bots_Observer_Collision_MN_VP_NAPF/Self Calculation 6/Neural network observer ==
  note: Update serial number
  note: Update serial number
  control_input : Inport
  x_agents : Inport  Port=2
  Finite observer : Subsystem
  Position selection : MATLAB Function  TreatAsAtomicUnit=on
  z_new : Outport
  z_used : Outport  Port=2
  wires:
  control_input/1 -> Finite observer/1(u)
  Position selection/1(x_agent) -> Finite observer/2(x)
  x_agents/1 -> Position selection/1(x_agents)
  Finite observer/1(z_new) -> z_new/1
  Finite observer/2(z_used) -> z_used/1

== system six_bots_Observer_Collision_MN_VP_NAPF/Self Calculation 6/Sliding mode differentiator ==
  note: Update serial number
  note: Update initial state
  Reference : Inport
  Integrator : Integrator  InitialCondition=[1.9;0.15;0;0;0;0;0;0;0;0;0;0]  ContinuousStateAttributes='speed'
  MATLAB Function : MATLAB Function  TreatAsAtomicUnit=on
  Reference selection : MATLAB Function  TreatAsAtomicUnit=on
  sliding mode differentiator : MATLAB Function  TreatAsAtomicUnit=on
  esti_references : Outport
  wires:
  Reference/1 -> Reference selection/1(reference)
  sliding mode differentiator/1(z_dot) -> Integrator/1
  MATLAB Function/1(esti_references) -> esti_references/1
  Reference selection/1(agent_reference) -> MATLAB Function/2(x_d), sliding mode differentiator/2(x_d)
  Integrator/1 -> MATLAB Function/1(z), sliding mode differentiator/1(z)

== system six_bots_Observer_Collision_MN_VP_NAPF/Self Calculation 6/Topology changing and APF ==
  note: Apply change here
  note: Update topology parameters
  note: Update APF parameter
  x_agents : Inport
  "Laplacian " : Inport  Port=2
  Changing topology : MATLAB Function  TreatAsAtomicUnit=on
  Communication based APF : MATLAB Function  TreatAsAtomicUnit=on
  rel_distance_6 : Scope
  F_i : Outport
  L_i : Outport  Port=2
  wires:
  x_agents/1 -> Communication based APF/1(x_agents), Changing topology/1(x_agents)
  "Laplacian "/1 -> Changing topology/2(L)
  Changing topology/1(rel_distance) -> rel_distance_6/1
  Changing topology/2(L_i) -> L_i/1, Communication based APF/2(L_i)
  Communication based APF/1(F_i) -> F_i/1

== system six_bots_Observer_Collision_MN_VP_NAPF/Self Calculation 1/Neural network observer/Finite observer ==
  note: Update serial number
  u : Inport
  x : Inport  Port=2
  Constant : Constant  Value=[0;0;0]
  Finite time observer : Subsystem  mask{z_hat_1=[1.5;0.4;0;0;0;0]}
      mask prompts: z_hat_1 "Simulink:blkprm_prompts:IntegratorInitCond"
      mask TypeOptions z_hat_1: z_hat_1/InitialCondition
      mask DialogControl z_hat_1 Prompt: Initial condition:
  Manual Switch : ManualSwitch  CurrentSetting=0
  Neural network : Subsystem
  Select useful information : MATLAB Function  TreatAsAtomicUnit=on
  z_hat : Scope
  z_new : Outport
  z_used : Outport  Port=2
  wires:
  Manual Switch/1 -> Finite time observer/1(f_hat), Select useful information/1(f_hat)
  Constant/1 -> Manual Switch/1
  Neural network/1(f_hat) -> Manual Switch/2
  u/1 -> Finite time observer/2(u)
  Finite time observer/1(z) -> Neural network/1(z), z_hat/1, Select useful information/2(z)
  Select useful information/1(z_new) -> z_new/1
  x/1 -> Select useful information/3(x), Finite time observer/3(x), Neural network/2(x)
  Select useful information/2(z_used) -> z_used/1

== system six_bots_Observer_Collision_MN_VP_NAPF/Self Calculation 2/Neural network observer/Finite observer ==
  note: Update serial number
  u : Inport
  x : Inport  Port=2
  Constant : Constant  Value=[0;0;0]
  Finite time observer : Subsystem  mask{z_hat_2=[-0.7;0.3;pi/4;0;0;0]}
      mask prompts: z_hat_2 "Simulink:blkprm_prompts:IntegratorInitCond"
      mask TypeOptions z_hat_2: z_hat_2/InitialCondition
      mask DialogControl z_hat_2 Prompt: Initial condition:
  Manual Switch : ManualSwitch  CurrentSetting=0
  Neural network : Subsystem
  Select useful information : MATLAB Function  TreatAsAtomicUnit=on
  z_hat : Scope
  z_new : Outport
  z_used : Outport  Port=2
  wires:
  Manual Switch/1 -> Finite time observer/1(f_hat), Select useful information/1(f_hat)
  Constant/1 -> Manual Switch/1
  Neural network/1(f_hat) -> Manual Switch/2
  u/1 -> Finite time observer/2(u)
  Finite time observer/1(z) -> Neural network/1(z), z_hat/1, Select useful information/2(z)
  Select useful information/1(z_new) -> z_new/1
  x/1 -> Neural network/2(x), Select useful information/3(x), Finite time observer/3(x)
  Select useful information/2(z_used) -> z_used/1

== system six_bots_Observer_Collision_MN_VP_NAPF/Self Calculation 3/Neural network observer/Finite observer ==
  note: Update serial number
  u : Inport
  x : Inport  Port=2
  Constant : Constant  Value=[0;0;0]
  Finite time observer : Subsystem  mask{z_hat_3=[-0.2;1.9;-pi/2;0;0;0]}
      mask prompts: z_hat_3 "Simulink:blkprm_prompts:IntegratorInitCond"
      mask TypeOptions z_hat_3: z_hat_3/InitialCondition
      mask DialogControl z_hat_3 Prompt: Initial condition:
  Manual Switch : ManualSwitch  CurrentSetting=0
  Neural network : Subsystem
  Select useful information : MATLAB Function  TreatAsAtomicUnit=on
  z_hat : Scope
  z_new : Outport
  z_used : Outport  Port=2
  wires:
  Manual Switch/1 -> Finite time observer/1(f_hat), Select useful information/1(f_hat)
  Constant/1 -> Manual Switch/1
  Neural network/1(f_hat) -> Manual Switch/2
  u/1 -> Finite time observer/2(u)
  Finite time observer/1(z) -> Neural network/1(z), z_hat/1, Select useful information/2(z)
  Select useful information/1(z_new) -> z_new/1
  x/1 -> Neural network/2(x), Select useful information/3(x), Finite time observer/3(x)
  Select useful information/2(z_used) -> z_used/1

== system six_bots_Observer_Collision_MN_VP_NAPF/Self Calculation 4/Neural network observer/Finite observer ==
  note: Update serial number
  u : Inport
  x : Inport  Port=2
  Constant : Constant  Value=[0;0;0]
  Finite time observer : Subsystem  mask{z_hat_4=[0.6;-0.3;7*pi/12;0;0;0]}
      mask prompts: z_hat_4 "Simulink:blkprm_prompts:IntegratorInitCond"
      mask TypeOptions z_hat_4: z_hat_4/InitialCondition
      mask DialogControl z_hat_4 Prompt: Initial condition:
  Manual Switch : ManualSwitch  CurrentSetting=0
  Neural network : Subsystem
  Select useful information : MATLAB Function  TreatAsAtomicUnit=on
  z_hat : Scope
  z_new : Outport
  z_used : Outport  Port=2
  wires:
  Manual Switch/1 -> Finite time observer/1(f_hat), Select useful information/1(f_hat)
  Constant/1 -> Manual Switch/1
  Neural network/1(f_hat) -> Manual Switch/2
  u/1 -> Finite time observer/2(u)
  Finite time observer/1(z) -> Neural network/1(z), z_hat/1, Select useful information/2(z)
  Select useful information/1(z_new) -> z_new/1
  x/1 -> Neural network/2(x), Select useful information/3(x), Finite time observer/3(x)
  Select useful information/2(z_used) -> z_used/1

== system six_bots_Observer_Collision_MN_VP_NAPF/Self Calculation 5/Neural network observer/Finite observer ==
  note: Update serial number
  u : Inport
  x : Inport  Port=2
  Constant : Constant  Value=[0;0;0]
  Finite time observer : Subsystem  mask{z_hat_5=[0;-1.1;pi/3;0;0;0]}
      mask prompts: z_hat_5 "Simulink:blkprm_prompts:IntegratorInitCond"
      mask TypeOptions z_hat_5: z_hat_5/InitialCondition
      mask DialogControl z_hat_5 Prompt: Initial condition:
  Manual Switch : ManualSwitch  CurrentSetting=0
  Neural network : Subsystem
  Select useful information : MATLAB Function  TreatAsAtomicUnit=on
  z_hat : Scope
  z_new : Outport
  z_used : Outport  Port=2
  wires:
  Manual Switch/1 -> Finite time observer/1(f_hat), Select useful information/1(f_hat)
  Constant/1 -> Manual Switch/1
  Neural network/1(f_hat) -> Manual Switch/2
  u/1 -> Finite time observer/2(u)
  Finite time observer/1(z) -> Neural network/1(z), z_hat/1, Select useful information/2(z)
  Select useful information/1(z_new) -> z_new/1
  x/1 -> Neural network/2(x), Select useful information/3(x), Finite time observer/3(x)
  Select useful information/2(z_used) -> z_used/1

== system six_bots_Observer_Collision_MN_VP_NAPF/Self Calculation 6/Neural network observer/Finite observer ==
  note: Update serial number
  u : Inport
  x : Inport  Port=2
  Constant : Constant  Value=[0;0;0]
  Finite time observer : Subsystem  mask{z_hat_6=[1.2;1.7;-pi/3;0;0;0]}
      mask prompts: z_hat_6 "Simulink:blkprm_prompts:IntegratorInitCond"
      mask TypeOptions z_hat_6: z_hat_6/InitialCondition
      mask DialogControl z_hat_6 Prompt: Initial condition:
  Manual Switch : ManualSwitch  CurrentSetting=0
  Neural network : Subsystem
  Select useful information : MATLAB Function  TreatAsAtomicUnit=on
  z_hat : Scope
  z_new : Outport
  z_used : Outport  Port=2
  wires:
  Manual Switch/1 -> Finite time observer/1(f_hat), Select useful information/1(f_hat)
  Constant/1 -> Manual Switch/1
  Neural network/1(f_hat) -> Manual Switch/2
  u/1 -> Finite time observer/2(u)
  Finite time observer/1(z) -> Neural network/1(z), z_hat/1, Select useful information/2(z)
  Select useful information/1(z_new) -> z_new/1
  x/1 -> Neural network/2(x), Select useful information/3(x), Finite time observer/3(x)
  Select useful information/2(z_used) -> z_used/1

== system six_bots_Observer_Collision_MN_VP_NAPF/Self Calculation 1/Neural network observer/Finite observer/Finite time observer ==
  note: Update serial number
  f_hat : Inport
  u : Inport  Port=2
  x : Inport  Port=3
  Initialisation : Subsystem
  Observer : MATLAB Function  TreatAsAtomicUnit=on
  x_tilde : Scope
  z_hat_1 : Integrator  InitialCondition=z_hat_1
  z : Outport
  wires:
  f_hat/1 -> Observer/1(f_hat)
  u/1 -> Initialisation/1(u_in)
  x/1 -> Observer/4(x)
  Observer/1(z_dot) -> z_hat_1/1
  Observer/2(x_tilde) -> x_tilde/1
  z_hat_1/1 -> Observer/2(z), z/1
  Initialisation/1(u_out) -> Observer/3(u)
